simulink model "CodeGenTest"  (R2019a)
settings: Solver=FixedStepDiscrete  StartTime=0.0  StopTime=10.0  RelTol=1e-3
model workspace (MATLAB code in the model file):
  | cmdLim = Simulink.Parameter;
  | cmdLim.Value = 15;
  | cmdLim.Description = 'Limit for controlling the maximum surface command angle.';
  | cmdLim.Min = 0;
  | cmdLim.Max = 90;
  | cmdLim.DocUnits = 'deg';
  | 
  | dispGain = Simulink.Parameter;
  | dispGain.Value = 0.75;
  | dispGain.Description = 'Gain applied to the displacement error.';
  | dispGain.Min = 0;
  | dispGain.Max = [];
  | dispGain.DocUnits = 'deg/sec/deg';
  | 
  | dispLim = Simulink.Parameter;
  | dispLim.Value = 30;
  | dispLim.Description = 'Limit for controlling the maximum commanded angle.';
  | dispLim.Min = 0;
  | dispLim.Max = 180;
  | dispLim.DocUnits = 'deg';
  | 
  | intGain = Simulink.Parameter;
  | intGain.Value = 0.5;
  | intGain.Description = 'Gain applied to the integral error.';
  | intGain.Min = 0;
  | intGain.Max = [];
  | intGain.DocUnits = 'deg/sec/deg/sec';
  | 
  | intLim = Simulink.Parameter;
  | intLim.Value = 5;
  | intLim.Description = 'Limit for controlling the maximum commanded angle.';
  | intLim.Min = 0;
  | intLim.Max = 90;
  | intLim.DocUnits = 'deg';
  | 
  | rateGain = Simulink.Parameter;
  | rateGain.Value = 2;
  | rateGain.Description = 'Gain applied to the rate error.';
  | rateGain.Min = 0;
  | rateGain.Max = [];
  | rateGain.DocUnits = 'deg/deg/sec';
  | 
  | rateLim = Simulink.Parameter;
  | rateLim.Value = 6;
  | rateLim.Description = 'Limit for controlling the maximum commanded angle.';
  | rateLim.Min = 0;
  | rateLim.Max = 180;
  | rateLim.DocUnits = 'deg/sec';
  | 
  | hdgGain = Simulink.Parameter;
  | hdgGain.Value = 0.015;
undefined symbols (not defined in the file or in its folder): fan_speed_type
libraries: simulink x1
settings Model: RequirementInfo={} %GIDa_fe9045fd_0412_4b6e_8206_617cc20e6fde  FPTRunName=Active  Creator=Derek  LastModifiedBy=Derek
settings SolverCC: AutoInsertRateTranBlk=on
settings DataIOCC: SaveOutput=off  SignalLogging=off  DSMLogging=off  SaveTime=off
settings OptimizationCC: DefaultParameterBehavior=Inlined  UseDivisionForNetSlopeComputation=on  GainParamInheritBuiltInType=on  UseFloatMulNetSlope=on  UseSpecifiedMinMax=on  InlineInvariantSignals=on  PassReuseOutputArgsAs=Individual arguments  ZeroExternalMemoryAtStartup=off  ZeroInternalMemoryAtStartup=off  NoFixptDivByZeroProtection=on  EfficientFloat2IntCast=on  LifeSpan=1  OptimizeBlockOrder=speed  DifferentSizesBufferReuse=on
settings DebuggingCC: SFUnexpectedBacktrackingDiag=warning  SFNoUnconditionalDefaultTransitionDiag=warning  SFExecutionAtInitializationDiag=none  ArithmeticOperatorsInVariantConditions=warning
settings HardwareCC: ProdBitPerPointer=32  ProdBitPerSizeT=32  ProdBitPerPtrDiffT=32  ProdLargestAtomicInteger=Long  ProdLargestAtomicFloat=Double  ProdWordSize=32  ProdLongLongMode=on  ProdHWDeviceType=ARM Compatible->ARM Cortex
settings SFSimCC: MATLABDynamicMemAlloc=off
settings RTWCC: SystemTargetFile=ert.tlc  GenCodeOnly=on  TemplateMakefile=ert_default_tmf  GenerateReport=on  BuildConfiguration=Faster Runs  IncludeHyperlinkInReport=on  LaunchReport=on  GenerateTraceInfo=on  GenerateTraceReport=on  GenerateTraceReportSl=on  GenerateTraceReportSf=on  GenerateTraceReportEml=on  GenerateCodeMetricsReport=on
settings CodeAppCC: GenerateComments=off  IgnoreCustomStorageClasses=off  OperatorAnnotations=on  SimulinkDataObjDesc=on  SFDataObjDesc=on  CustomSymbolStrGlobalVar=$N$M  CustomSymbolStrType=$N$M  CustomSymbolStrFcn=$N$M$F  CustomSymbolStrBlkIO=$N$M  CustomSymbolStrMacro=$N$M  InsertBlockDesc=on  EnableCustomComments=on  ReqsInCode=on
settings ERTTargetCC: TargetLangStandard=C99 (ISO)  UtilityFuncGeneration=Shared location  MultiwordLength=2048  IncludeMdlTerminateFcn=off  CombineSignalStateStructs=on  SuppressErrorStatus=on  SupportAbsoluteTime=off  PurelyIntegerCode=on  SupportNonFinite=off  SupportComplex=off  InlinedParameterPlacement=NonHierarchical  ERTCustomFileTemplate=example_file_process.tlc  ERTFilePackagingFormat=CompactWithDataFile  PreserveIfCondition=on  ConvertIfToSwitch=off
settings ConfigComp: CovScope=ReferencedModels  CovSaveName=covdata_rollAP  CovMetricSettings=dcmtrwe  CovHTMLOptions=-sRT=1 -aTS=1 -bRG=1 -bTC=1 -hTR=1 -nFC=0 -scm=1 -bcm=1 -xEv=0  CovSaveCumulativeToWorkspaceVar=on  CovSaveSingleToWorkspaceVar=on  CovCumulativeVarName=covCumulativeData_rollAP  CovReportOnPause=off  CovExternalEMLEnable=off  CovSFcnEnable=off

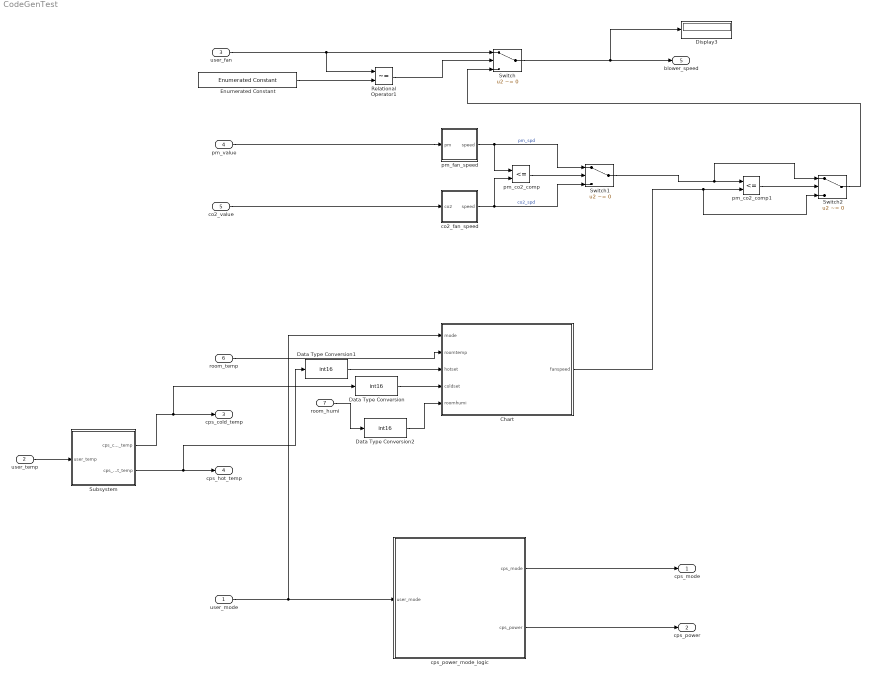
== system CodeGenTest ==
  user_mode : Inport  OutDataTypeStr=Enum: user_mode_type
  user_temp : Inport  Port=2  OutDataTypeStr=uint16
  user_fan : Inport  Port=3  OutDataTypeStr=Enum: fan_speed_type
  pm_value : Inport  Port=4  OutDataTypeStr=uint16
  co2_value : Inport  Port=5  OutDataTypeStr=uint16
  room_temp : Inport  Port=6  OutDataTypeStr=int16
  room_humi : Inport  Port=7  OutDataTypeStr=uint16
  Chart : Stateflow chart  BlockKeywords=__PRM__SERIALIZED__DATA__:Stateflow Chart,Stateflow Diagram  TreatAsAtomicUnit=on
  Data Type Conversion : DataTypeConversion  OutDataTypeStr=int16
  Data Type Conversion1 : DataTypeConversion  OutDataTypeStr=int16
  Data Type Conversion2 : DataTypeConversion  OutDataTypeStr=int16
  Display3 : Display
  Enumerated Constant : simulink/Sources/Enumerated Constant  OutDataTypeStr=Enum: fan_speed_type  Value=fan_speed_type.fan_speed_auto  SampleTime=inf
      settings: SourceProductName=Simulink
  Relational Operator1 : RelationalOperator  Operator=~=  OutDataTypeStr=boolean  RndMeth=Simplest
  Subsystem : Subsystem
  Switch : Switch  Criteria=u2 ~= 0  OutDataTypeStr=Enum: fan_speed_type
  Switch1 : Switch  Criteria=u2 ~= 0  OutDataTypeStr=Enum: fan_speed_type
  Switch2 : Switch  Criteria=u2 ~= 0  OutDataTypeStr=Enum: fan_speed_type
  co2_fan_speed : Stateflow chart  BlockKeywords=__PRM__SERIALIZED__DATA__:Stateflow Chart,Stateflow Diagram  TreatAsAtomicUnit=on
  "cps_power_mode_logic " : Stateflow chart  BlockKeywords=__PRM__SERIALIZED__DATA__:Stateflow Chart,Stateflow Diagram  TreatAsAtomicUnit=on
  pm_co2_comp : RelationalOperator  Operator=<=  OutDataTypeStr=boolean  RndMeth=Simplest
  pm_co2_comp1 : RelationalOperator  Operator=<=  OutDataTypeStr=boolean  RndMeth=Simplest
  pm_fan_speed : Stateflow chart  BlockKeywords=__PRM__SERIALIZED__DATA__:Stateflow Chart,Stateflow Diagram  TreatAsAtomicUnit=on
  cps_mode : Outport  OutDataTypeStr=Enum: cps_mode_type
  "cps_power " : Outport  Port=2  OutDataTypeStr=Enum: cps_power_type
  cps_cold_temp : Outport  Port=3
  cps_hot_temp : Outport  Port=4
  "blower_speed " : Outport  Port=5
  wires:
  user_mode/1 -> Chart/1(mode), "cps_power_mode_logic "/1(user_mode)
  "cps_power_mode_logic "/1(cps_mode) -> cps_mode/1
  "cps_power_mode_logic "/2(cps_power) -> "cps_power "/1
  user_fan/1 -> Relational Operator1/1, Switch/1
  Switch/1 -> Display3/1, "blower_speed "/1
  pm_value/1 -> pm_fan_speed/1(pm)
  co2_value/1 -> co2_fan_speed/1(co2)
  Relational Operator1/1 -> Switch/2
  Enumerated Constant/1 -> Relational Operator1/2
  pm_fan_speed/1(speed) -> Switch1/1, pm_co2_comp/1  "pm_spd"
  co2_fan_speed/1(speed) -> Switch1/3, pm_co2_comp/2  "co2_spd"
  pm_co2_comp/1 -> Switch1/2
  user_temp/1 -> Subsystem/1(user_temp)
  Subsystem/1(cps_cold_temp) -> Data Type Conversion/1, cps_cold_temp/1
  Subsystem/2(cps_hot_temp) -> Data Type Conversion1/1, cps_hot_temp/1
  room_temp/1 -> Chart/2(roomtemp)
  room_humi/1 -> Data Type Conversion2/1
  Chart/1(fanspeed) -> Switch2/3, pm_co2_comp1/2
  Data Type Conversion1/1 -> Chart/3(hotset)
  Data Type Conversion/1 -> Chart/4(coldset)
  Data Type Conversion2/1 -> Chart/5(roomhumi)
  Switch1/1 -> Switch2/1, pm_co2_comp1/1
  pm_co2_comp1/1 -> Switch2/2
  Switch2/1 -> Switch/3

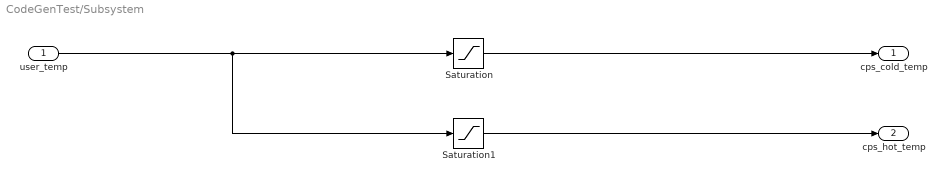
== system CodeGenTest/Subsystem ==
  user_temp : Inport  OutDataTypeStr=uint16
  Saturation : Saturate  UpperLimit=300  LowerLimit=120
  Saturation1 : Saturate  UpperLimit=360  LowerLimit=180
  cps_cold_temp : Outport
  cps_hot_temp : Outport  Port=2
  wires:
  Saturation1/1 -> cps_hot_temp/1
  user_temp/1 -> Saturation1/1, Saturation/1
  Saturation/1 -> cps_cold_temp/1

== stateflow chart CodeGenTest/pm_fan_speed ==
  settings: updateMethod=DISCRETE  sampleTime=0.1
  state low
    en:speed=fan_speed_low;
    du:speed=fan_speed_low;
  state silent
    entry: speed=fan_speed_silent;
    du: speed=fan_speed_silent;
  state mid
    en:speed=fan_speed_mid;
    du:speed=fan_speed_mid;
  state high
    en:speed=fan_speed_high;
    du:speed=fan_speed_high;
  (default) -> silent
  silent -> low : [pm>=35]
  low -> mid [order 1] : [pm>=75]
  mid -> high [order 1] : [pm>=150]
  mid -> low [order 2] : [pm<70]
  low -> silent [order 2] : [pm<30 &&  after(5,sec)]
  high -> mid : [pm<145]
  data: pm input; speed output Enum: fan_speed_type

== stateflow chart CodeGenTest/Chart ==
  state speed=cal_temp_speed(diff) [function]
    (default) -> (junction 55) : % cal_temp_speed_logic
    (junction 55) -> (junction 56) [order 1] : [diff>=5]
    (junction 55) -> (junction 57) [order 2]
    (junction 56) -> (junction 64) : {speed=fan_speed_type.fan_speed_high;}
    (junction 57) -> (junction 58) [order 1] : [diff<5 && diff>=3]
    (junction 57) -> (junction 59) [order 2]
    (junction 58) -> (junction 63) : {speed=fan_speed_type.fan_speed_mid;}
    (junction 59) -> (junction 60) [order 1] : [diff<3 && diff>=1]
    (junction 59) -> (junction 61) [order 2] : {speed=fan_speed_type.fan_speed_silent;}
    (junction 60) -> (junction 62) : {speed=fan_speed_type.fan_speed_low;}
    (junction 62) -> (junction 61)
    (junction 63) -> (junction 62)
    (junction 64) -> (junction 63)
    (junction 61) -> (junction 65)
  state speed=cal_humi_speed(humi) [function]
    (default) -> (junction 90) : % cal_humi_speed_logic
    (junction 90) -> (junction 91) [order 1] : [humi>=80]
    (junction 90) -> (junction 92) [order 2]
    (junction 91) -> (junction 78) : {speed=fan_speed_type.fan_speed_high;}
    (junction 92) -> (junction 79) [order 1] : [humi<80 && humi>=70]
    (junction 92) -> (junction 80) [order 2]
    (junction 79) -> (junction 76) : {speed=fan_speed_type.fan_speed_mid;}
    (junction 80) -> (junction 73) [order 1] : [humi<70 && humi>=60]
    (junction 80) -> (junction 74) [order 2] : {speed=fan_speed_type.fan_speed_silent;}
    (junction 73) -> (junction 75) : {speed=fan_speed_type.fan_speed_low;}
    (junction 75) -> (junction 74)
    (junction 76) -> (junction 75)
    (junction 78) -> (junction 76)
    (junction 74) -> (junction 77)
  (default) -> (junction 23)
  (junction 23) -> (junction 25) [order 1] : [mode==user_mode_cold]{tempdiff=roomtemp-coldset;}
  (junction 23) -> (junction 27) [order 2]
  (junction 25) -> (junction 66) : {fanspeed=cal_temp_speed(tempdiff);}
  (junction 27) -> (junction 29) [order 1] : [mode==user_mode_hot]{tempdiff=hotset-roomtemp;}
  (junction 27) -> (junction 31) [order 2]
  (junction 29) -> (junction 68) : {fanspeed=cal_temp_speed(tempdiff);}
  (junction 31) -> (junction 33) [order 1] : [mode==user_mode_dehumi]{fanspeed=cal_humi_speed(roomhumi);}
  (junction 31) -> (junction 102) [order 2] : {fanspeed=fan_speed_silent;}
  (junction 33) -> (junction 98)
  (junction 98) -> (junction 102)
  (junction 68) -> (junction 98)
  (junction 66) -> (junction 68)
  (junction 102) -> (junction 105)
  data: diff function_input; speed function_output; humi function_input; speed function_output; mode input Enum: user_mode_type; roomtemp input int16; hotset input int16; coldset input int16; fanspeed output Enum: fan_speed_type; tempdiff local int16; roomhumi input int16

== stateflow chart CodeGenTest/cps_power_mode_logic  ==
  (default) -> (junction 122) : % cpslogic
  (junction 122) -> (junction 123) [order 1] : [user_mode==user_mode_auto]
  (junction 122) -> (junction 124) [order 2]
  (junction 123) -> (junction 131) : {cps_power=cps_power_on;cps_mode=cps_mode_auto;}
  (junction 124) -> (junction 125) [order 1] : [user_mode==user_mode_cold]
  (junction 124) -> (junction 126) [order 2]
  (junction 125) -> (junction 130) : {cps_power=cps_power_on;cps_mode=cps_mode_cold;}
  (junction 126) -> (junction 127) [order 1] : [user_mode==user_mode_hot]
  (junction 126) -> (junction 133) [order 2]
  (junction 127) -> (junction 129) : {cps_power=cps_power_on;cps_mode=cps_mode_hot;}
  (junction 133) -> (junction 135) [order 1] : [user_mode==user_mode_dehumi]
  (junction 133) -> (junction 128) [order 2] : {cps_power=cps_power_off;}
  (junction 135) -> (junction 136) : {cps_power=cps_power_on;cps_mode=cps_mode_dehumi;}
  (junction 136) -> (junction 128)
  (junction 129) -> (junction 136)
  (junction 130) -> (junction 129)
  (junction 131) -> (junction 130)
  (junction 128) -> (junction 132)
  data: user_mode input Enum: user_mode_type; cps_mode output Enum: cps_mode_type [-40..80]; cps_power output Enum: cps_power_type

== stateflow chart CodeGenTest/co2_fan_speed ==
  state low
    en:speed=fan_speed_low;
    du:speed=fan_speed_low;
  state silent
    en:speed=fan_speed_silent;
    du:speed=fan_speed_silent;
  state mid
    en:speed=fan_speed_mid;
    du:speed=fan_speed_mid;
  state high
    en:speed=fan_speed_high;
    du:speed=fan_speed_high;
  (default) -> silent
  silent -> low : [co2>=600]
  low -> mid [order 1] : [co2>=1000]
  mid -> high [order 1] : [co2>=1400]
  mid -> low [order 2] : [co2<980]
  low -> silent [order 2] : [co2<580]
  high -> mid : [co2<1380]
  data: co2 input; speed output Enum: fan_speed_type
